simulink model "boostObserverR2017a"  (R2017a)
settings: Solver=VariableStepAuto  StartTime=0.0  StopTime=1.5  FixedStep=0.0005  EnableMultiTasking=on
InitFcn:
  | kp=0.01;
  | ki=0.01;
  | 
  | k=2;
  | em=100000000;
  | GE=1/em;
  | GU=k*ki/GE;
  | GCE=k*kp/GU;
model workspace (MAT data in the model file):
  time = 0.8
values from neighbouring files (symbols this model uses):
  A1 = obj.boostConverter.A1    [BoostController.m]    (also in BoostConverter.m = [-obj.R/obj.L 0;0 -1/(obj.Ro*obj.C)]; BuckBoostConverter.m = [-obj.R/obj.L 0;0 -1/(obj.Ro*obj.C)]; obsmc.m = Asigma{1,1}; workspace_atual.mat = [-16.4  0; 0  -3.50877192982])
  A2 = obj.boostConverter.A2    [BoostController.m]    (also in BoostConverter.m = [-obj.R/obj.L -1/obj.L;1/obj.C -1/(obj.Ro*obj.C)]; BuckBoostConverter.m = [-obj.R/obj.L 1/obj.L;-1/obj.C -1/(obj.Ro*obj.C)]; obsmc.m = Asigma{1,2}; workspace_atual.mat = [-16.4  -200; 350.877192982  -3.50877192982])
  B1 = obj.boostConverter.B1    [BoostController.m]    (also in BoostConverter.m = [1/obj.L;0]; BuckBoostConverter.m = [1/obj.L;0]; obsmc.m = Bsigma{1,1}; workspace_atual.mat = [200 0])
  Cmatrix = [1  0; 0  1]    [workspace_atual.mat]    (also in workspace_certo.mat)
  rho = 5    [workspace_atual.mat]    (also in workspace_certo.mat)
  RMSfrequency = 47.61    [BoostFaultSimulation.m]    (also in workspace_atual.mat; workspace_certo.mat)
  Smep = 80    [workspace_atual.mat]    (also in workspace_certo.mat)
  ueq = 0.5    [workspace_atual.mat]    (also in workspace_certo.mat)
  x_e = [ie;ve]    [BoostConverter.m]    (also in BuckBoostConverter.m)
  xe = obj.boostConverter.equilibriumstate(ve)    [BoostController.m]    (also in workspace_atual.mat = [7.62509288104 380]; workspace_certo.mat = [7.62509288104 380])
undefined symbols (not defined in the file or in its folder): Atilde1, Atilde2, Ctilde1, Dtilde1, Dtilde2, F, G
undefined symbols (not defined in the file): R, Ro
libraries: powerlib_meascontrol x1, PhdLibrary x1, dspmtrx3 x1, dspstat3 x1, simulink x1, dspmathops x1, powerlib x1
settings Model: SimulationMode=accelerator  Creator=d13go  LastModifiedBy=d13go
settings SolverCC: MaxConsecutiveZCs=10000  ZeroCrossAlgorithm=Adaptive
settings DataIOCC: SaveFinalState=on  SaveState=on  ReturnWorkspaceOutputs=on  LoggingToFile=on
settings OptimizationCC: DefaultParameterBehavior=Inlined  UseDivisionForNetSlopeComputation=on  UseFloatMulNetSlope=on  InlineInvariantSignals=on  EfficientFloat2IntCast=on  LifeSpan=1
settings DebuggingCC: ReadBeforeWriteMsg=DisableAll  WriteAfterWriteMsg=DisableAll  WriteAfterReadMsg=DisableAll  AlgebraicLoopMsg=error  MaxConsecutiveZCsMsg=warning  MaskedZcDiagnostic=none  IgnoredZcDiagnostic=none  MultiTaskDSMMsg=none  SFUnexpectedBacktrackingDiag=warning  SFNoUnconditionalDefaultTransitionDiag=warning
settings HardwareCC: ProdLongLongMode=on
settings ModelReferenceCC: UpdateModelReferenceTargets=IfOutOfDate
settings SFSimCC: SFSimEcho=off  MATLABDynamicMemAlloc=off
settings RTWCC: GenerateReport=on  LaunchReport=on
settings CodeAppCC: ForceParamTrailComments=on
settings GRTTargetCC: TargetLangStandard=C89/C90 (ANSI)  CombineSignalStateStructs=on  MatFileLogging=off  SupportVariableSizeSignals=on
settings ConfigComp: CovMetricSettings=dw  CovHtmlReporting=on  CovSaveCumulativeToWorkspaceVar=on  CovSaveSingleToWorkspaceVar=on  CovExternalEMLEnable=off
settings SimscapeCC: SimscapeNormalizeSystem=off

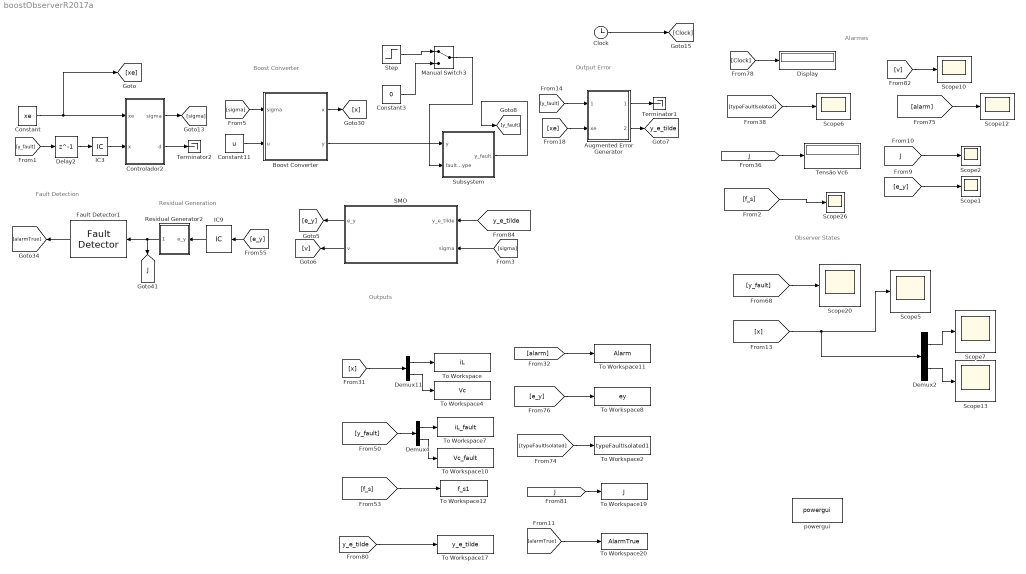
== system boostObserverR2017a ==
  note: Alarmes
  note: Observer States
  note: Residual Generation
  note: Fault Detection
  note: Boost Converter
  note: Output Error
  note: Outputs
  Augmented Error Generator : Subsystem  mask{Cmatrix=Cmatrix, Ctilde1=Ctilde1}
      mask prompts: Cmatrix "Output Matrix"; Ctilde1 "Output matrix augmented:"
  Boost Converter : Subsystem  mask(Boots State-Space model){A1=A1, A2=A2, B1=B1, R=R, Ro=Ro, Cmatrix=Cmatrix}
      mask prompts: A1 "A1 matrix"; A2 "A2 matrix"; B1 "B matrix"; R "Resistance"; Ro "Output Resistance"; Cmatrix "Output Matrix"
      mask help: Boots State-Space model
      mask Display: disp('Boost')
  Clock : Clock
  Constant : Constant  Value=xe  VectorParams1D=off
  Constant11 : Constant  Value=u
  Constant3 : Constant  Value=0
  Controlador2 : Subsystem  mask(Sliding mode controller){KiVc=2.3, KVc=0.2, ueq=ueq, Smep=Smep, KiL=2, Freq=7000}
      mask prompts: KiVc "Integral voltage gain"; KVc "Voltage gain"; ueq "Equilibrium signal"; Smep "Surface limit layer"; KiL "Current gain"; Freq "Frequency"
      mask help: Sliding mode controller with integral for boost converter
  Delay2 : Delay  DelayLength=1
  Demux11 : Demux  Outputs=2
  Demux2 : Demux  Outputs=2
  Demux4 : Demux  Outputs=2
  Display : Display
  Fault Detector1 : PhdLibrary/Fault Detector  Jth=0
      settings: SourceProductName=Phd Diego
  IC3 : InitialCondition  Value=[0;0]
  IC9 : InitialCondition  Value=[0;0]
  Manual Switch3 : ManualSwitch
  Residual Generator2 : Subsystem  mask{RMSfrequency=RMSfrequency/10}
      mask prompts: RMSfrequency "Windows length:"
      mask help: RMS generator for two dimensios
  SMO : Subsystem  mask(Sliding mode observer){G=G, F=F, Atilde1=Atilde1, Atilde2=Atilde2, Dtilde1=Dtilde1, Dtilde2=Dtilde2, Ctilde1=Ctilde1, rho=rho}
      mask prompts: G "G matrix"; F "F matrix"; Atilde1 "A1 matrix augmented"; Atilde2 "A2 matrix augmented"; Dtilde1 "D1 matrix augmented"; Dtilde2 "D2 matrix augmented"; Ctilde1 "C1 matrix augmented"; rho "Sliding surface coefficient (rho)"
      mask help: Sligin mode observer for fault detection in switched affine linear systems
      mask Help: Enter the system matrices and the observer gains
      mask Display: disp('\dot{x} = Ax + b \\ y = Cx','texmode','on');
  Scope{1..2,5..7,10,12..13,20,26} (10 alike) : Scope
  Step : Step  Time=0.70  SampleTime=0
  Subsystem : Subsystem  mask(Step faults){iLfgain=20, Vcfgain=20}
      mask prompts: iLfgain "Current fault gain (A)"; Vcfgain "Voltage fault gain (V)"
      mask help: Configure a step fault
  Tensão Vc6 : Display
  Terminator1 : Terminator
  Terminator2 : Terminator
  To Workspace : ToWorkspace  VariableName=iL  SaveFormat=Timeseries  SampleTime=-1
  To Workspace10 : ToWorkspace  VariableName=Vc_fault  SaveFormat=Timeseries  SampleTime=-1
  To Workspace11 : ToWorkspace  VariableName=Alarm  SaveFormat=Timeseries  SampleTime=-1
  To Workspace12 : ToWorkspace  VariableName=f_s1  SaveFormat=Timeseries  SampleTime=-1
  To Workspace17 : ToWorkspace  VariableName=y_e_tilde  SaveFormat=Timeseries  SampleTime=-1
  To Workspace19 : ToWorkspace  VariableName=J  SaveFormat=Timeseries  SampleTime=-1
  To Workspace2 : ToWorkspace  VariableName=typeFaultIsolated1  SaveFormat=Timeseries  SampleTime=-1
  To Workspace20 : ToWorkspace  VariableName=AlarmTrue  SaveFormat=Timeseries  SampleTime=-1
  To Workspace4 : ToWorkspace  VariableName=Vc  SaveFormat=Timeseries  SampleTime=-1
  To Workspace7 : ToWorkspace  VariableName=iL_fault  SaveFormat=Timeseries  SampleTime=-1
  To Workspace8 : ToWorkspace  VariableName=ey  SaveFormat=Timeseries  SampleTime=-1
  powergui : powerlib/powergui  Priority=1  SimulationMode=Discrete  SampleTime=50e-6  frequency=60  Iterations=50  frequencyindice=0  Pbase=100e6  ErrMax=1e-4  UnitsV=kV  UnitsW=MW  buscounter=0  FunctionMessages=off  echomessages=off  EnableUseOfTLC=off  CurrentSourceSwitches=off  DisableSnubberDevices=off  DisableRonSwitches=off  DisableVfSwitches=off  DisplayEquations=off  AutomaticDiscreteSolvers=off  SolverType=Tustin/Backward Euler (TBE)  Interpol=off  ExternalGateDelay=off  methode=off  Ts=100  x0status=blocks  SPID=on  SwTol=0  HookPort=off  NonlinearTolerance=1e-4  nMaxIteration=100  ContinueOnMaxIteration=off  RestoreLinks=warning  ResistiveCurrentMeasurement=off  Frange=[0:2:500]  Ylog=off  Xlog=on  ShowGrid=off  save=off  variable=ZData  structure=0  ZoomFFT=off  StartTime=0.0  cycles=1  DisplayStyle=1  fundamental=60  FreqAxis=off  MaxFrequency=1000  frequencyindicesteady=1  RmsSteady=1  display=off
  tag scope: J=global, y_e_tilde=global
  wires:
  [y_fault] -> Scope20/1
  Clock/1 -> [Clock]
  IC9/1 -> Residual Generator2/1(e_y)
  [x] -> Demux2/1, Scope5/1
  Boost Converter/1(x) -> [x]
  [f_s] -> Scope26/1
  Augmented Error Generator/1(e_tilde) -> Terminator1/1
  [alarm] -> To Workspace11/1
  Augmented Error Generator/2(y_e_tilde) -> [y_e_tilde]
  Controlador2/2(d) -> Terminator2/1
  Boost Converter/2(y) -> Subsystem/1(y)
  [y_e_tilde] -> SMO/1(y_e_tilde)
  Subsystem/1(y_fault) -> [y_fault]
  [xe] -> Augmented Error Generator/2(xe)
  [y_e_tilde] -> To Workspace17/1
  Demux11/1 -> To Workspace/1
  Demux11/2 -> To Workspace4/1
  IC3/1 -> Controlador2/2(x)
  Residual Generator2/1(RMS) -> Fault Detector1/1, [J]
  Step/1 -> Manual Switch3/1
  Demux4/2 -> To Workspace10/1
  Constant/1 -> [xe], Controlador2/1(xe)
  [y_fault] -> Augmented Error Generator/1(y_fault)
  Fault Detector1/1 -> [alarmTrue]
  Delay2/1 -> IC3/1
  [sigma] -> SMO/2(sigma)
  [Clock] -> Display/1
  SMO/2(v) -> [v]
  [e_y] -> IC9/1
  SMO/1(e_y) -> [e_y]
  [e_y] -> To Workspace8/1
  Constant3/1 -> Manual Switch3/2
  Controlador2/1(sigma) -> [sigma]
  [x] -> Demux11/1
  Constant11/1 -> Boost Converter/2(u)
  [f_s] -> To Workspace12/1
  [sigma] -> Boost Converter/1(sigma)
  [alarmTrue] -> To Workspace20/1
  Demux2/2 -> Scope13/1
  [v] -> Scope10/1
  [e_y] -> Scope1/1
  Manual Switch3/1 -> Subsystem/2(faultType)
  [J] -> To Workspace19/1
  Demux2/1 -> Scope7/1
  [typeFaultIsolated] -> To Workspace2/1
  [J] -> Scope2/1
  [alarm] -> Scope12/1
  [J] -> Tensão Vc6/1
  [y_fault] -> Delay2/1
  [y_fault] -> Demux4/1
  Demux4/1 -> To Workspace7/1
  [typeFaultIsolated] -> Scope6/1

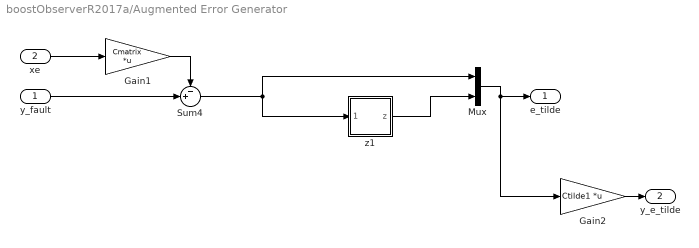
== system boostObserverR2017a/Augmented Error Generator ==
  y_fault : Inport
  xe : Inport  Port=2
  Gain1 : Gain  Gain=Cmatrix  Multiplication=Matrix(K*u)
  Gain2 : Gain  Gain=Ctilde1  Multiplication=Matrix(K*u)
  Mux : Mux  Inputs=2
  Sum4 : Sum  Inputs=-+|
  z1 : Subsystem
  e_tilde : Outport
  y_e_tilde : Outport  Port=2
  wires:
  z1/1(z) -> Mux/2
  Mux/1 -> Gain2/1, e_tilde/1
  Gain2/1 -> y_e_tilde/1
  xe/1 -> Gain1/1
  Gain1/1 -> Sum4/1
  y_fault/1 -> Sum4/2
  Sum4/1 -> Mux/1, z1/1(z_dot)

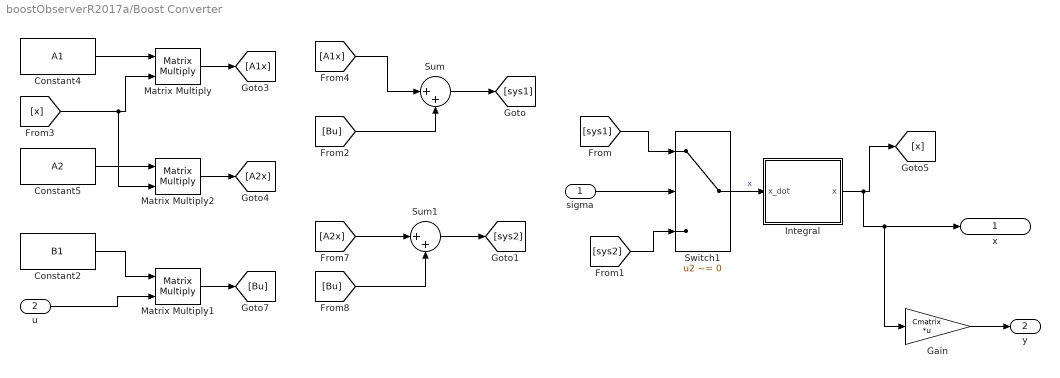
== system boostObserverR2017a/Boost Converter ==
  sigma : Inport
  u : Inport  Port=2
  Constant2 : Constant  Value=B1  VectorParams1D=off
  Constant4 : Constant  Value=A1  VectorParams1D=off
  Constant5 : Constant  Value=A2  VectorParams1D=off
  Gain : Gain  Gain=Cmatrix  Multiplication=Matrix(K*u)
  Integral : Subsystem
  Matrix Multiply : Product  Multiplication=Matrix(*)
  Matrix Multiply1 : Product  Multiplication=Matrix(*)
  Matrix Multiply2 : Product  Multiplication=Matrix(*)
  Sum : Sum  Inputs=|++
  Sum1 : Sum  Inputs=|++
  Switch1 : Switch  Criteria=u2 ~= 0
  x : Outport
  y : Outport  Port=2
  wires:
  [A1x] -> Sum/1
  [x] -> Matrix Multiply2/2, Matrix Multiply/2
  [Bu] -> Sum1/2
  [Bu] -> Sum/2
  Constant5/1 -> Matrix Multiply2/1
  Constant4/1 -> Matrix Multiply/1
  Matrix Multiply2/1 -> [A2x]
  [sys1] -> Switch1/1
  Matrix Multiply/1 -> [A1x]
  Sum/1 -> [sys1]
  Sum1/1 -> [sys2]
  [sys2] -> Switch1/3
  Switch1/1 -> Integral/1(x_dot)  "x"
  [A2x] -> Sum1/1
  sigma/1 -> Switch1/2
  Constant2/1 -> Matrix Multiply1/1
  Matrix Multiply1/1 -> [Bu]
  u/1 -> Matrix Multiply1/2
  Integral/1(x) -> Gain/1, x/1, [x]
  Gain/1 -> y/1

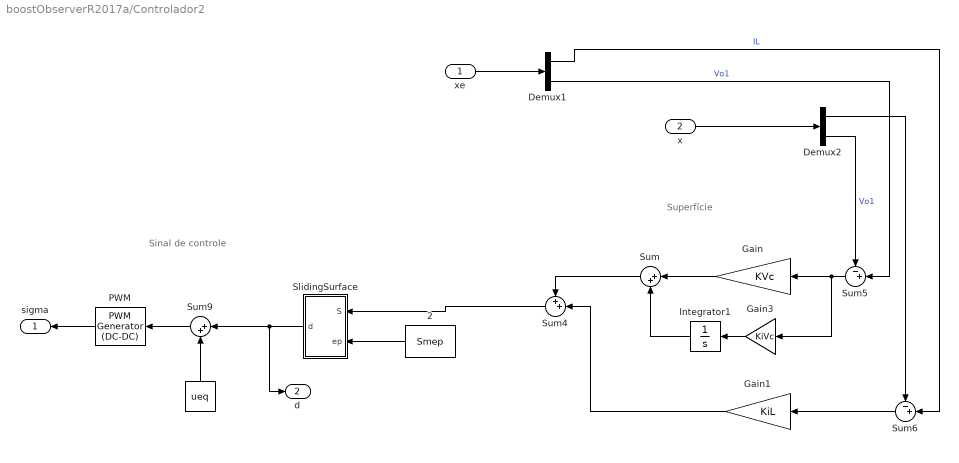
== system boostObserverR2017a/Controlador2 ==
  note: Sinal de controle
  note: Superfície
  xe : Inport
  x : Inport  Port=2
  "    " : Constant  Value=ueq
  "    2" : Constant  Value=Smep
  Demux1 : Demux  Outputs=2
  Demux2 : Demux  Outputs=2
  Gain : Gain  Gain=KVc
  Gain1 : Gain  Gain=KiL
  Gain3 : Gain  Gain=KiVc
  Integrator1 : Integrator
  PWM : powerlib_meascontrol/Pulse & Signal Generators/PWM Generator (DC-DC)  Fsw=Freq  Ts=0
  SlidingSurface : Subsystem
  Sum : Sum  Inputs=|++
  Sum4 : Sum  Inputs=++|
  Sum5 : Sum  Inputs=-+|
  Sum6 : Sum  Inputs=-+|
  Sum9 : Sum  Inputs=|++
  sigma : Outport
  d : Outport  Port=2
  wires:
  Demux1/1 -> Sum6/2  "IL"
  PWM/1 -> sigma/1
  Demux2/2 -> Sum5/1  "Vo1"
  "    "/1 -> Sum9/2
  Sum5/1 -> Gain3/1, Gain/1
  Sum9/1 -> PWM/1
  Demux1/2 -> Sum5/2  "Vo1"
  Demux2/1 -> Sum6/1
  x/1 -> Demux2/1
  Gain1/1 -> Sum4/2
  Gain/1 -> Sum/1
  Sum/1 -> Sum4/1
  SlidingSurface/1(d) -> d/1, Sum9/1
  "    2"/1 -> SlidingSurface/2(ep)
  Sum6/1 -> Gain1/1
  Gain3/1 -> Integrator1/1
  Sum4/1 -> SlidingSurface/1(S)
  Integrator1/1 -> Sum/2
  xe/1 -> Demux1/1

== system boostObserverR2017a/Residual Generator2 ==
  e_y : Inport
  Matrix Square1 : dspmtrx3/Matrix Square  OutMin=[]  OutMax=[]
      settings: SourceProductBaseCode=DS
  Moving RMS : dspstat3/Moving RMS  Method=Sliding window  SpecifyWindowLength=on  WindowLength=RMSfrequency/10  ForgettingFactor=0.9  SimulateUsing=Code generation
      settings: SourceProductBaseCode=DS
  Sqrt2 : Sqrt  SaturateOnIntegerOverflow=on
  RMS : Outport
  wires:
  Matrix Square1/1 -> Sqrt2/1
  Sqrt2/1 -> Moving RMS/1
  Moving RMS/1 -> RMS/1
  e_y/1 -> Matrix Square1/1

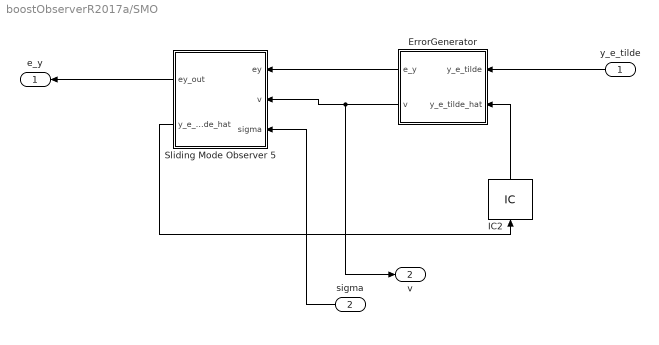
== system boostObserverR2017a/SMO ==
  y_e_tilde : Inport
  sigma : Inport  Port=2
  ErrorGenerator : Subsystem
  IC2 : InitialCondition  Value=[0;0]
  Sliding Mode Observer 5 : Subsystem
  e_y : Outport
  v : Outport  Port=2
  wires:
  Sliding Mode Observer 5/1(ey_out) -> e_y/1
  Sliding Mode Observer 5/2(y_e_tilde_hat) -> IC2/1
  ErrorGenerator/2(v) -> v/1, Sliding Mode Observer 5/2(v)
  ErrorGenerator/1(e_y) -> Sliding Mode Observer 5/1(ey)
  IC2/1 -> ErrorGenerator/2(y_e_tilde_hat)
  y_e_tilde/1 -> ErrorGenerator/1(y_e_tilde)
  sigma/1 -> Sliding Mode Observer 5/3(sigma)

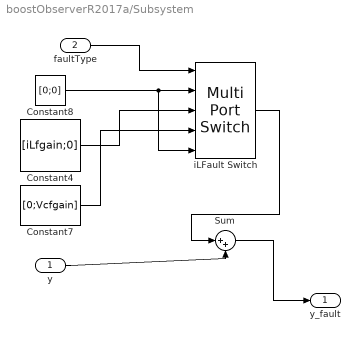
== system boostObserverR2017a/Subsystem ==
  y : Inport
  faultType : Inport  Port=2
  Constant4 : Constant  Value=[iLfgain;0]  VectorParams1D=off
  Constant7 : Constant  Value=[0;Vcfgain]  VectorParams1D=off
  Constant8 : Constant  Value=[0;0]  VectorParams1D=off
  Sum : Sum  Inputs=|++
  iLFault Switch : MultiPortSwitch  DataPortOrder=Zero-based contiguous  DataPortForDefault=Additional data port  zeroidx=on
  y_fault : Outport
  wires:
  y/1 -> Sum/2
  Constant8/1 -> iLFault Switch/5, iLFault Switch/2
  iLFault Switch/1 -> Sum/1
  Constant7/1 -> iLFault Switch/4
  Constant4/1 -> iLFault Switch/3
  faultType/1 -> iLFault Switch/1
  Sum/1 -> y_fault/1

== system boostObserverR2017a/Augmented Error Generator/z1 ==
  z_dot : Inport
  Constant1 : Constant  Value=[0;0]  VectorParams1D=off
  Gain2 : Gain  Gain=Cmatrix  Multiplication=Matrix(K*u) (u vector)
  Integrator6 : Integrator  InitialConditionSource=external
  z : Outport
  wires:
  Gain2/1 -> Integrator6/1
  Integrator6/1 -> z/1
  z_dot/1 -> Gain2/1
  Constant1/1 -> Integrator6/2

== system boostObserverR2017a/Boost Converter/Integral ==
  x_dot : Inport
  Ground : Ground
  Ground1 : Ground
  IC : InitialCondition  Value=[0;0]
  Integrator1 : Integrator  InitialConditionSource=external  InitialCondition=[-x_e; 0; 0]
  Mux : Mux  Inputs=2
  x : Outport
  wires:
  x_dot/1 -> Integrator1/1
  Integrator1/1 -> x/1
  IC/1 -> Integrator1/2
  Ground1/1 -> Mux/2
  Ground/1 -> Mux/1
  Mux/1 -> IC/1

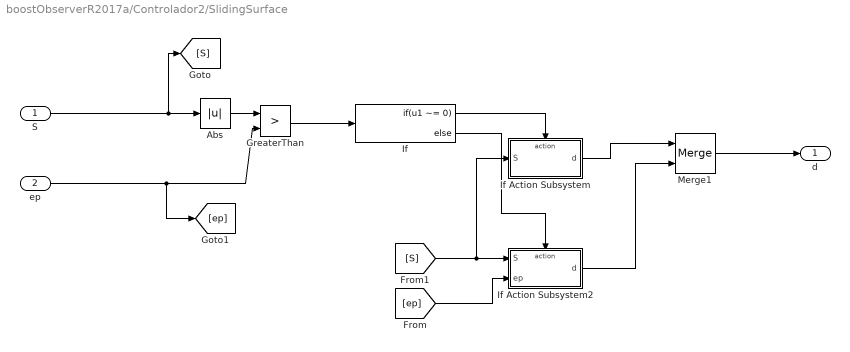
== system boostObserverR2017a/Controlador2/SlidingSurface ==
  S : Inport
  ep : Inport  Port=2
  Abs : Abs
  GreaterThan : RelationalOperator  Operator=>  OutDataTypeStr=boolean  RndMeth=Simplest
  If : If  IfExpression=u1 ~= 0
  If Action Subsystem : Subsystem  TreatAsAtomicUnit=on
  If Action Subsystem2 : Subsystem  TreatAsAtomicUnit=on
  Merge1 : Merge
  d : Outport
  wires:
  If Action Subsystem2/1(d) -> Merge1/2
  [S] -> If Action Subsystem/1(S), If Action Subsystem2/1(S)
  If/2 -> If Action Subsystem2/Action
  If/1 -> If Action Subsystem/Action
  [ep] -> If Action Subsystem2/2(ep)
  S/1 -> [S], Abs/1
  If Action Subsystem/1(d) -> Merge1/1
  Abs/1 -> GreaterThan/1
  GreaterThan/1 -> If/1
  Merge1/1 -> d/1
  ep/1 -> [ep], GreaterThan/2

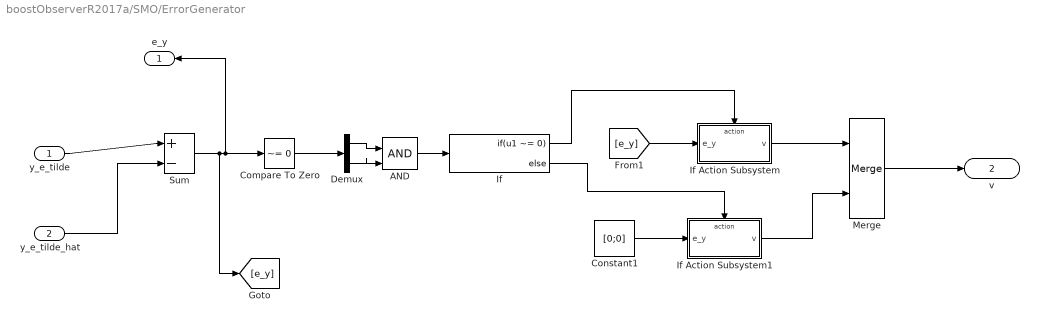
== system boostObserverR2017a/SMO/ErrorGenerator ==
  y_e_tilde : Inport
  y_e_tilde_hat : Inport  Port=2
  AND : Logic  IconShape=distinctive  AllPortsSameDT=off  OutDataTypeStr=boolean
  Compare To Zero : simulink/Logic and Bit Operations/Compare To Zero  relop=~=  OutDataTypeStr=boolean
  Constant1 : Constant  Value=[0;0]
  Demux : Demux  Outputs=2
  If : If  IfExpression=u1 ~= 0
  If Action Subsystem : Subsystem  TreatAsAtomicUnit=on
  If Action Subsystem1 : Subsystem  TreatAsAtomicUnit=on
  Merge : Merge  InitialOutput=[0;0]
  Sum : Sum  Inputs=|+-
  e_y : Outport
  v : Outport  Port=2
  wires:
  y_e_tilde/1 -> Sum/1
  y_e_tilde_hat/1 -> Sum/2
  Sum/1 -> Compare To Zero/1, e_y/1, [e_y]
  If/1 -> If Action Subsystem/Action
  If/2 -> If Action Subsystem1/Action
  [e_y] -> If Action Subsystem/1(e_y)
  Constant1/1 -> If Action Subsystem1/1(e_y)
  If Action Subsystem/1(v) -> Merge/1
  If Action Subsystem1/1(v) -> Merge/2
  Demux/1 -> AND/1
  Demux/2 -> AND/2
  AND/1 -> If/1
  Merge/1 -> v/1
  Compare To Zero/1 -> Demux/1

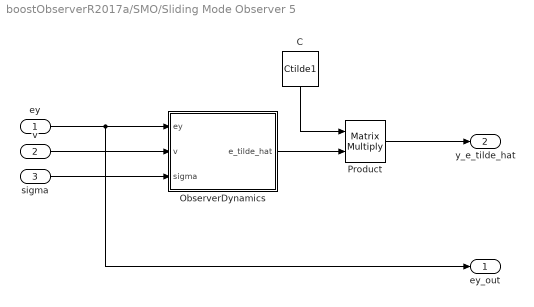
== system boostObserverR2017a/SMO/Sliding Mode Observer 5 ==
  ey : Inport
  v : Inport  Port=2
  sigma : Inport  Port=3
  C : Constant  Value=Ctilde1
  ObserverDynamics : Subsystem
  Product : Product  Multiplication=Matrix(*)
  ey_out : Outport
  y_e_tilde_hat : Outport  Port=2
  wires:
  Product/1 -> y_e_tilde_hat/1
  C/1 -> Product/1
  ObserverDynamics/1(e_tilde_hat) -> Product/2
  sigma/1 -> ObserverDynamics/3(sigma)
  ey/1 -> ey_out/1, ObserverDynamics/1(ey)
  v/1 -> ObserverDynamics/2(v)

== system boostObserverR2017a/Controlador2/SlidingSurface/If Action Subsystem ==
  S : Inport
  Action Port : ActionPort
  Sign : Signum
  d : Outport
  wires:
  S/1 -> Sign/1
  Sign/1 -> d/1

== system boostObserverR2017a/Controlador2/SlidingSurface/If Action Subsystem2 ==
  S : Inport
  ep : Inport  Port=2
  Action Port : ActionPort
  Divide : Product  Inputs=*/
  d : Outport
  wires:
  S/1 -> Divide/1
  ep/1 -> Divide/2
  Divide/1 -> d/1

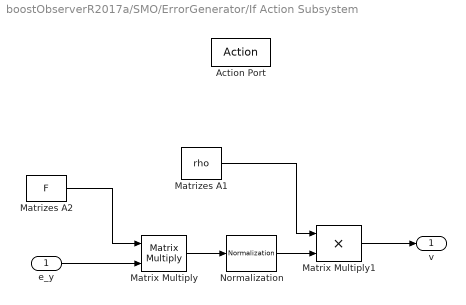
== system boostObserverR2017a/SMO/ErrorGenerator/If Action Subsystem ==
  e_y : Inport
  Action Port : ActionPort
  Matrix Multiply : Product  Multiplication=Matrix(*)
  Matrix Multiply1 : Product
  Matrizes A1 : Constant  Value=rho
  Matrizes A2 : Constant  Value=F  VectorParams1D=off
  Normalization : dspmathops/Normalization  NormType=2-norm  Bias=1e-10  NormOver=Each column  Dimension=1  roundingMode=Floor  overflowMode=off  accumDataTypeStr=Inherit: Same as product output  accumLastDataTypeStr=Inherit: Same as product output  outputDataTypeStr=Inherit: Same as product output  outputMin=[]  outputMax=[]  outputLastDataTypeStr=Inherit: Same as product output
  v : Outport
  wires:
  Matrix Multiply/1 -> Normalization/1
  Matrizes A2/1 -> Matrix Multiply/1
  Normalization/1 -> Matrix Multiply1/2
  e_y/1 -> Matrix Multiply/2
  Matrizes A1/1 -> Matrix Multiply1/1
  Matrix Multiply1/1 -> v/1

== system boostObserverR2017a/SMO/ErrorGenerator/If Action Subsystem1 ==
  e_y : Inport
  Action Port : ActionPort
  v : Outport
  wires:
  e_y/1 -> v/1

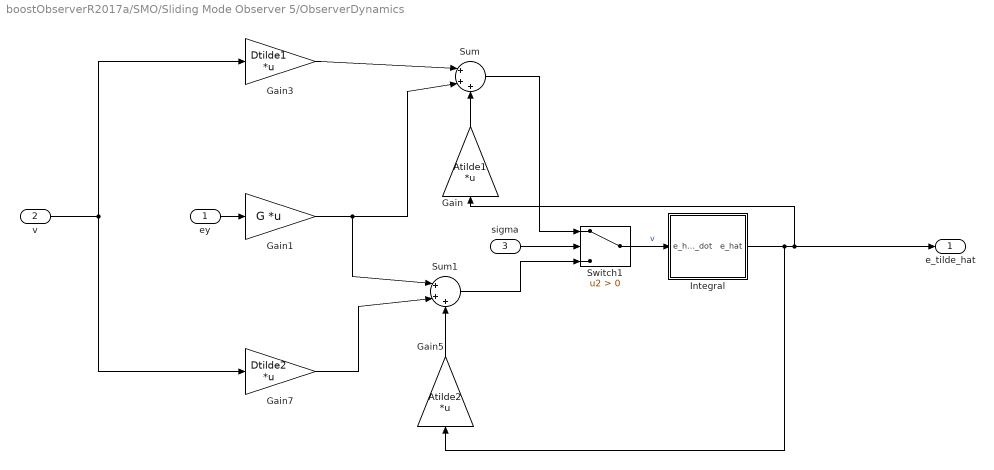
== system boostObserverR2017a/SMO/Sliding Mode Observer 5/ObserverDynamics ==
  ey : Inport
  v : Inport  Port=2
  sigma : Inport  Port=3
  Gain : Gain  Gain=Atilde1  Multiplication=Matrix(K*u)
  Gain1 : Gain  Gain=G  Multiplication=Matrix(K*u)
  Gain3 : Gain  Gain=Dtilde1  Multiplication=Matrix(K*u)
  Gain5 : Gain  Gain=Atilde2  Multiplication=Matrix(K*u)
  Gain7 : Gain  Gain=Dtilde2  Multiplication=Matrix(K*u)
  Integral : Subsystem
  Sum : Sum  Inputs=|+++
  Sum1 : Sum  Inputs=|+++
  Switch1 : Switch  Criteria=u2 > Threshold
  e_tilde_hat : Outport
  wires:
  sigma/1 -> Switch1/2
  Switch1/1 -> Integral/1(e_hat_dot)  "v"
  Integral/1(e_hat) -> Gain/1, e_tilde_hat/1, Gain5/1
  ey/1 -> Gain1/1
  v/1 -> Gain7/1, Gain3/1
  Sum1/1 -> Switch1/3
  Sum/1 -> Switch1/1
  Gain7/1 -> Sum1/2
  Gain5/1 -> Sum1/3
  Gain3/1 -> Sum/1
  Gain1/1 -> Sum1/1, Sum/2
  Gain/1 -> Sum/3

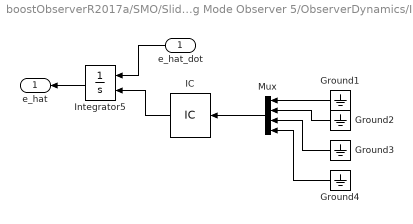
== system boostObserverR2017a/SMO/Sliding Mode Observer 5/ObserverDynamics/Integral ==
  e_hat_dot : Inport
  Ground{1..4} (4 alike) : Ground
  IC : InitialCondition  Value=[-xe;0;0]
  Integrator5 : Integrator  InitialConditionSource=external  InitialCondition=[-x_e; 0; 0]
  Mux : Mux
  e_hat : Outport
  wires:
  e_hat_dot/1 -> Integrator5/1
  Integrator5/1 -> e_hat/1
  IC/1 -> Integrator5/2
  Ground1/1 -> Mux/1
  Ground2/1 -> Mux/2
  Ground3/1 -> Mux/3
  Ground4/1 -> Mux/4
  Mux/1 -> IC/1
